simulink model "simulinkzad1"  (R2013b)
settings: Solver=ode45  StartTime=0.0  StopTime=10.0  RelTol=1e-3
values from neighbouring files (symbols this model uses):
  czasProbki = 0.25    [Zadanie1wersjaSimulink.m]
  populacja = 25    [Zadanie1wersjaSimulink.m]    (also in Zadanie2.m = x; na zajeciach.m = x)
  wspolczynnik = 1.2    [Zadanie1wersjaSimulink.m]
  wspolczynnikCiagly = -1    [Zadanie1wersjaSimulink.m]
undefined symbols (not defined in the file or in its folder): iloscProbek
libraries: simulink x1
settings Model: Creator=Jonatan  LastModifiedBy=Jonatan

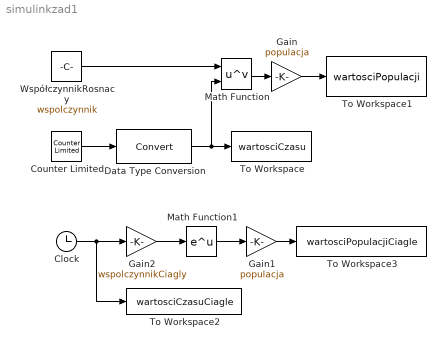
== system simulinkzad1 ==
  Clock : Clock
  Counter Limited : simulink/Sources/Counter Limited  uplimit=iloscProbek  tsamp=czasProbki
  Data Type Conversion : DataTypeConversion  SampleTime=czasProbki
  Gain : Gain  Gain=populacja  SampleTime=czasProbki
  Gain1 : Gain  Gain=populacja
  Gain2 : Gain  Gain=wspolczynnikCiagly
  Math Function : Math  Operator=pow  SampleTime=czasProbki  SaturateOnIntegerOverflow=on
  Math Function1 : Math  SaturateOnIntegerOverflow=on
  To Workspace : ToWorkspace  VariableName=wartosciCzasu  SampleTime=czasProbki
  To Workspace1 : ToWorkspace  VariableName=wartosciPopulacji  SampleTime=czasProbki
  To Workspace2 : ToWorkspace  VariableName=wartosciCzasuCiagle  SampleTime=-1
  To Workspace3 : ToWorkspace  VariableName=wartosciPopulacjiCiagle  SampleTime=-1
  WspółczynnikRosnacy : Constant  Value=wspolczynnik
  wires:
  Math Function/1 -> Gain/1
  WspółczynnikRosnacy/1 -> Math Function/1
  Gain/1 -> To Workspace1/1
  Counter Limited/1 -> Data Type Conversion/1
  Data Type Conversion/1 -> Math Function/2, To Workspace/1
  Clock/1 -> Gain2/1, To Workspace2/1
  Gain1/1 -> To Workspace3/1
  Math Function1/1 -> Gain1/1
  Gain2/1 -> Math Function1/1
